simulink model "linetrack_"  (Simulink 7.3)
settings: Solver=ode23t  StartTime=0.0  StopTime=10  RelTol=1e-3
libraries: simulink x1
settings Model: Creator=Sainquake  LastModifiedBy=Sainquake Notebook
settings SolverCC: MaxConsecutiveZCs=10000  ZeroCrossAlgorithm=Adaptive

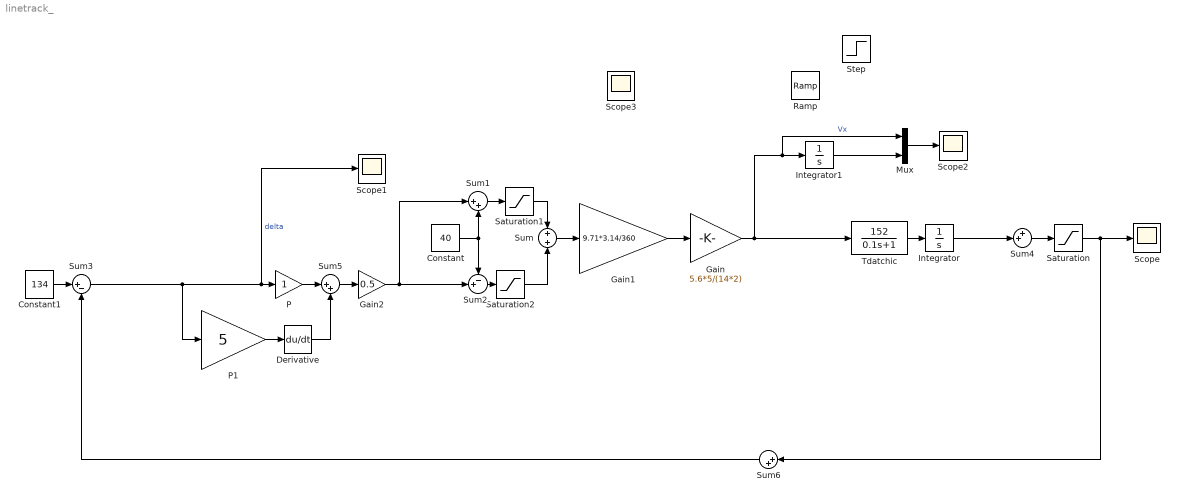
== system linetrack_ ==
  Constant : Constant  Value=40  OutDataType=fixdt(1, 16)  OutScaling=2^0
  Constant1 : Constant  Value=134  OutDataType=fixdt(1, 16)  OutScaling=2^0
  Derivative : Derivative
  Gain : Gain  Gain=5.6*5/(14*2)  ParameterDataType=fixdt(1, 16)  ParameterScaling=2^0  OutDataType=fixdt(1, 16)  OutScaling=2^0
  Gain1 : Gain  Gain=9.71*3.14/360  ParameterDataType=fixdt(1, 16)  ParameterScaling=2^0  OutDataType=fixdt(1, 16)  OutScaling=2^0
  Gain2 : Gain  Gain=0.5  ParameterDataType=fixdt(1, 16)  ParameterScaling=2^0  OutDataType=fixdt(1, 16)  OutScaling=2^0
  Integrator : Integrator
  Integrator1 : Integrator
  Mux : Mux  Inputs=2
  P : Gain  ParameterDataType=fixdt(1, 16)  ParameterScaling=2^0  OutDataType=fixdt(1, 16)  OutScaling=2^0
  P1 : Gain  Gain=5  ParameterDataType=fixdt(1, 16)  ParameterScaling=2^0  OutDataType=fixdt(1, 16)  OutScaling=2^0
  Ramp : simulink/Sources/Ramp  SystemSampleTime=-1  slope=10  start=0  X0=0
  Saturation : Saturate  UpperLimit=210  LowerLimit=58  OutDataType=fixdt(1, 16)  OutScaling=2^0
  Saturation1 : Saturate  UpperLimit=100  LowerLimit=-100  OutDataType=fixdt(1, 16)  OutScaling=2^0
  Saturation2 : Saturate  UpperLimit=100  LowerLimit=-100  OutDataType=fixdt(1, 16)  OutScaling=2^0
  Scope{,1..3} (4 alike) : Scope
      Scope1 settings: YMax=65
      Scope2 settings: SaveName=ScopeData2
      Scope3 settings: SaveName=ScopeData3
  Step : Step  After=152  SampleTime=0  ZeroCross=off
  Sum : Sum  Inputs=+|+  OutDataType=fixdt(1, 16)  OutScaling=2^0
  Sum1 : Sum  Inputs=|++  OutDataType=fixdt(1, 16)  OutScaling=2^0
  Sum2 : Sum  Inputs=-+|  OutDataType=fixdt(1, 16)  OutScaling=2^0
  Sum3 : Sum  Inputs=|+-  OutDataType=fixdt(1, 16)  OutScaling=2^0
  Sum4 : Sum  Inputs=++|  OutDataType=fixdt(1, 16)  OutScaling=2^0
  Sum5 : Sum  Inputs=|++  OutDataType=fixdt(1, 16)  OutScaling=2^0
  Sum6 : Sum  Inputs=|++  OutDataType=fixdt(1, 16)  OutScaling=2^0
  Tdatchic : TransferFcn  Numerator=[152]  Denominator=[0.1 1]
  wires:
  Sum/1 -> Gain1/1
  Gain1/1 -> Gain/1
  Constant/1 -> Sum2/1, Sum1/2
  Sum1/1 -> Saturation1/1
  Sum2/1 -> Saturation2/1
  Gain2/1 -> Sum2/2, Sum1/1
  Constant1/1 -> Sum3/1
  Sum3/1 -> Scope1/1, P/1, P1/1  "delta"
  Gain/1 -> Integrator1/1, Mux/1, Tdatchic/1  "Vx"
  P/1 -> Sum5/1
  ? -> Sum4/1
  Saturation/1 -> Scope/1, Sum6/1
  Sum4/1 -> Saturation/1
  Sum5/1 -> Gain2/1
  Derivative/1 -> Sum5/2
  P1/1 -> Derivative/1
  Saturation1/1 -> Sum/1
  Saturation2/1 -> Sum/2
  Sum6/1 -> Sum3/2
  ? -> Sum6/2
  Integrator1/1 -> Mux/2
  Mux/1 -> Scope2/1
  Tdatchic/1 -> Integrator/1
  Integrator/1 -> Sum4/2
